simulink model "FuzzyPidCtrl"  (R2016b)
settings: Solver=VariableStepAuto  StartTime=0.0  StopTime=20  RelTol=1e-3
libraries: fuzblock x1
settings Model: Creator=Polonsky  LastModifiedBy=Polonsky

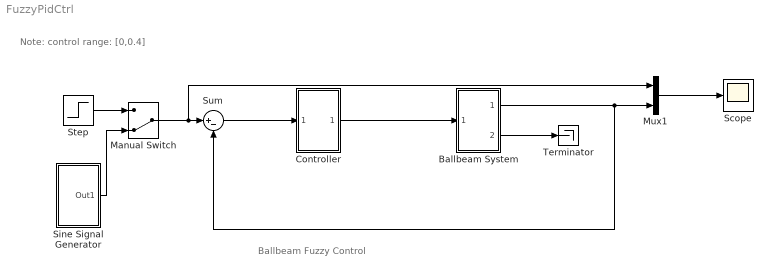
== system FuzzyPidCtrl ==
  note: Note: control range: [0,0.4]
  note: Ballbeam Fuzzy Control
  Ballbeam System : Subsystem
  Controller : Subsystem
  Manual Switch : ManualSwitch  CurrentSetting=0
  Mux1 : Mux  Inputs=2
  Scope : Scope
  Sine Signal Generator : Subsystem  mask{Amplitude=0.2, Frequency=0.2}
      mask prompts: Amplitude "Amplitude of refernece signal"; Frequency "Frequency of reference signal"
  Step : Step  After=0.2  SampleTime=0
  Sum : Sum  Inputs=|+-
  Terminator : Terminator
  wires:
  Mux1/1 -> Scope/1
  Ballbeam System/1(position) -> Sum/2, Mux1/2
  Manual Switch/1 -> Mux1/1, Sum/1
  Step/1 -> Manual Switch/1
  Sine Signal Generator/1(Out1) -> Manual Switch/2
  Sum/1 -> Controller/1(In1)
  Controller/1(Out1) -> Ballbeam System/1(In1)
  Ballbeam System/2(velocity) -> Terminator/1

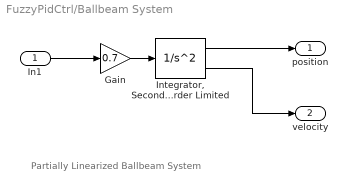
== system FuzzyPidCtrl/Ballbeam System ==
  note: Partially Linearized Ballbeam System
  In1 : Inport
  Gain : Gain  Gain=0.7
  "Integrator, Second-Order Limited" : SecondOrderIntegrator  ICX=0  LimitX=on  UpperLimitX=0.4  LowerLimitX=0
  position : Outport
  velocity : Outport  Port=2
  wires:
  Gain/1 -> "Integrator, Second-Order Limited"/1
  In1/1 -> Gain/1
  "Integrator, Second-Order Limited"/2 -> velocity/1
  "Integrator, Second-Order Limited"/1 -> position/1

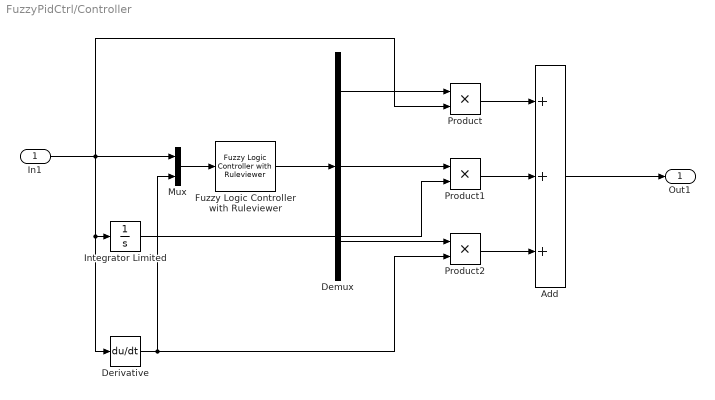
== system FuzzyPidCtrl/Controller ==
  In1 : Inport
  Add : Sum  Inputs=+++
  Demux : Demux  Outputs=3
  Derivative : Derivative
  Fuzzy Logic Controller with Ruleviewer : fuzblock/Fuzzy Logic  Controller  with Ruleviewer  fismatrix=Fuzzy_PID_Controller  Ts=2
  Integrator Limited : Integrator  LimitOutput=on  UpperSaturationLimit=1  LowerSaturationLimit=0
  Mux : Mux  Inputs=2
  Product : Product
  Product1 : Product
  Product2 : Product
  Out1 : Outport
  wires:
  Product/1 -> Add/1
  In1/1 -> Derivative/1, Integrator Limited/1, Mux/1, Product/2
  Fuzzy Logic Controller with Ruleviewer/1 -> Demux/1
  Demux/1 -> Product/1
  Demux/2 -> Product1/1
  Demux/3 -> Product2/1
  Mux/1 -> Fuzzy Logic Controller with Ruleviewer/1
  Derivative/1 -> Mux/2, Product2/2
  Integrator Limited/1 -> Product1/2
  Product1/1 -> Add/2
  Product2/1 -> Add/3
  Add/1 -> Out1/1

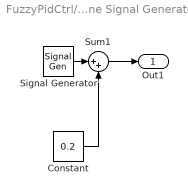
== system FuzzyPidCtrl/Sine Signal Generator ==
  Constant : Constant  Value=0.2
  Signal Generator : SignalGenerator  Amplitude=Amplitude  Frequency=Frequency  Units=rad/sec
  Sum1 : Sum  Inputs=|++
  Out1 : Outport
  wires:
  Constant/1 -> Sum1/2
  Sum1/1 -> Out1/1
  Signal Generator/1 -> Sum1/1
